simulink model "SVpwm2L_block_level"  (R2023b)
settings: Solver=FixedStepAuto  StartTime=0.0  StopTime=0.1  FixedStep=1e-5  RelTol=1e-4  EnableMultiTasking=on
libraries: spsIGBTDiodeLib x6, spsSeriesRLCBranchLib x3, spsVoltageMeasurementLib x2, spsDCVoltageSourceLib x1, spsGroundLib x1, simulink x1, spsThreePhaseVIMeasurementLib x1, sps_lib x1
settings Model: Creator=Ranit  LastModifiedBy=hhp
settings SolverCC: AlgebraicLoopSolver=TrustRegion
settings DataIOCC: ReturnWorkspaceOutputs=off
settings OptimizationCC: LifeSpan=inf
settings DebuggingCC: UnconnectedInputMsg=warning  UnconnectedOutputMsg=warning  UnconnectedLineMsg=warning  SFUnexpectedBacktrackingDiag=warning  SFNoUnconditionalDefaultTransitionDiag=warning  ArithmeticOperatorsInVariantConditions=warning
settings ModelReferenceCC: EnableRefExpFcnMdlSchedulingChecks=on
settings SFSimCC: SimUseLocalCustomCode=off  CustomCodeUndefinedFunction=UseInterfaceOnly
settings RTWCC: RTWUseLocalCustomCode=off
settings CodeAppCC: StateflowObjectComments=on
settings GRTTargetCC: TargetLangStandard=C89/C90 (ANSI)
settings ConfigComp: CovMetricSettings=dw  CovSaveCumulativeToWorkspaceVar=on  CovSaveSingleToWorkspaceVar=on  CovExternalEMLEnable=off
settings SimscapeCC: SimscapeNormalizeSystem=off

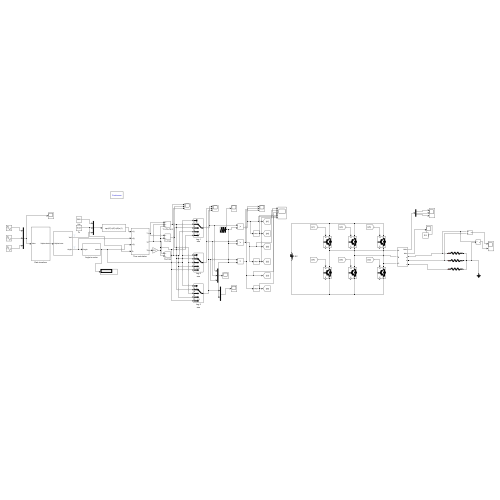
[thumbnail: Simulink's stored preview of the top-level diagram]
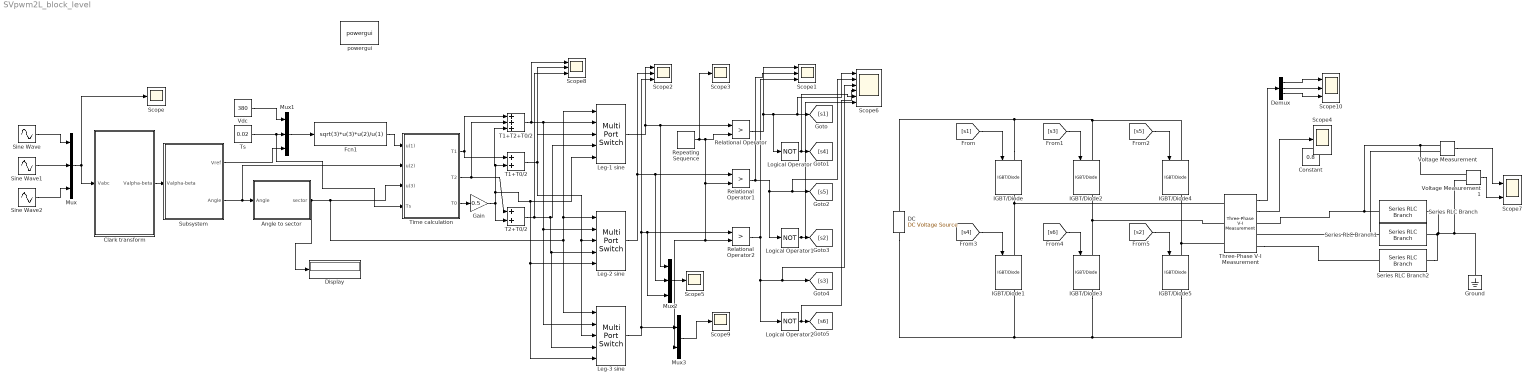
== system SVpwm2L_block_level ==
  Angle to sector : Subsystem
  Clark transform : Subsystem
  Constant : Constant  Value=0.8
  "DC " : spsDCVoltageSourceLib/DC Voltage Source  Amplitude=400  Measurements=None
  Demux : Demux  Outputs=3
  Display : Display
  Fcn1 : Fcn  Expr=sqrt(3)*u(3)*u(2)/u(1)
  Gain : Gain  Gain=0.5
  Ground : spsGroundLib/Ground  LConnTagsString=a
  IGBT/Diode{,1..5} (6 alike) : spsIGBTDiodeLib/IGBT//Diode  Ron=1e-3  Rs=1e5  Cs=inf  Measurements=on
  Leg-1 sine : MultiPortSwitch  DataPortOrder=Specify indices  Inputs=4  DataPortIndices={[1,6],2,5,[3,4]}  SaturateOnIntegerOverflow=off  InputSameDT=off
  Leg-2 sine : MultiPortSwitch  DataPortOrder=Specify indices  Inputs=4  DataPortIndices={[2,3],4,1,[5,6]}  SaturateOnIntegerOverflow=off  InputSameDT=off
  Leg-3 sine : MultiPortSwitch  DataPortOrder=Specify indices  Inputs=4  DataPortIndices={[4,5],6,3,[1,2]}  SaturateOnIntegerOverflow=off  InputSameDT=off
  Logical Operator : Logic  Operator=NOT  AllPortsSameDT=off  OutDataTypeStr=boolean
  Logical Operator1 : Logic  Operator=NOT  AllPortsSameDT=off  OutDataTypeStr=boolean
  Logical Operator2 : Logic  Operator=NOT  AllPortsSameDT=off  OutDataTypeStr=boolean
  Mux : Mux  Inputs=3
  Mux1 : Mux  Inputs=3
  Mux2 : Mux  Inputs=3
  Mux3 : Mux  Inputs=2
  Relational Operator : RelationalOperator  Operator=>  OutDataTypeStr=boolean  InputSameDT=off
  Relational Operator1 : RelationalOperator  Operator=>  OutDataTypeStr=boolean  InputSameDT=off
  Relational Operator2 : RelationalOperator  Operator=>  OutDataTypeStr=boolean  InputSameDT=off
  Repeating Sequence : simulink/Sources/Repeating Sequence  rep_seq_t=[0 1]*[1/3000]  rep_seq_y=[0 0.03]
  Scope{,3..5,9} (5 alike) : Scope
  Scope{1..2,8,10} (4 alike) : Scope  NumInputPorts=3
  Scope6 : Scope  NumInputPorts=6
  Scope7 : Scope  NumInputPorts=2
  Series RLC Branch : spsSeriesRLCBranchLib/Series RLC Branch  LConnTagsString=__new0  RConnTagsString=__new0  BranchType=R  Resistance=5  Inductance=1e-3  SetiL0=off  InitialCurrent=0  Capacitance=1e-6  Setx0=off  InitialVoltage=0  Measurements=None
  Series RLC Branch1 : spsSeriesRLCBranchLib/Series RLC Branch  LConnTagsString=__new0  RConnTagsString=__new0  BranchType=R  Resistance=5  Inductance=1e-3  SetiL0=off  InitialCurrent=0  Capacitance=1e-6  Setx0=off  InitialVoltage=0  Measurements=None
  Series RLC Branch2 : spsSeriesRLCBranchLib/Series RLC Branch  LConnTagsString=__new0  RConnTagsString=__new0  BranchType=R  Resistance=5  Inductance=1e-3  SetiL0=off  InitialCurrent=0  Capacitance=1e-6  Setx0=off  InitialVoltage=0  Measurements=None
  Sine Wave : Sin  Amplitude=230  Frequency=2*pi*50  SampleTime=0
  Sine Wave1 : Sin  Amplitude=230  Frequency=2*pi*50  Phase=2*pi/3  SampleTime=0
  Sine Wave2 : Sin  Amplitude=230  Frequency=2*pi*50  Phase=4*pi/3  SampleTime=0
  Subsystem : Subsystem
  T1+T0/2 : Sum
  T1+T2+T0/2 : Sum  Inputs=+++
  T2+T0/2 : Sum
  Three-Phase V-I Measurement : spsThreePhaseVIMeasurementLib/Three-Phase V-I Measurement  VoltageMeasurement=phase-to-phase  SetLabelV=off  LabelV=Vabc  Vpu=off  VpuLL=off  CurrentMeasurement=yes  SetLabelI=off  LabelI=Iabc  Ipu=off  Pbase=100e6  Vbase=500e3  OutputType=Complex  PhasorSimulation=off  PSBequivalent=0
  Time calculation : Subsystem
  Ts : Constant  Value=0.02
  Vdc : Constant  Value=380
  Voltage Measurement : spsVoltageMeasurementLib/Voltage Measurement  PhasorSimulation=off  OutputType=Complex  PSBequivalent=0
  Voltage Measurement1 : spsVoltageMeasurementLib/Voltage Measurement  PhasorSimulation=off  OutputType=Complex  PSBequivalent=0
  powergui : sps_lib/powergui  Priority=1  SimulationMode=Continuous  SampleTime=10e-6  frequency=60  Iterations=50  frequencyindice=0  Pbase=100e6  ErrMax=1e-4  UnitsV=kV  UnitsW=MW  buscounter=0  FunctionMessages=off  echomessages=off  EnableUseOfTLC=off  CurrentSourceSwitches=on  DisableSnubberDevices=off  DisableRonSwitches=off  DisableVfSwitches=off  DisplayEquations=off  AutomaticDiscreteSolvers=off  SolverType=Tustin/Backward Euler (TBE)  Interpol=off  ExternalGateDelay=off  methode=off  Ts=10  x0status=blocks  SPID=off  SwTol=0  HookPort=off  NonlinearTolerance=1e-4  nMaxIteration=100  ContinueOnMaxIteration=off  RestoreLinks=warning  ResistiveCurrentMeasurement=off  Frange=[0:2:500]  Ylog=off  Xlog=on  ShowGrid=off  save=off  variable=ZData  structure=ScopeData1  ZoomFFT=off  StartTime=0.0  cycles=1  DisplayStyle=1  fundamental=50  FreqAxis=off  MaxFrequency=1000  frequencyindicesteady=1  RmsSteady=1  display=off
  wires:
  Sine Wave1/1 -> Mux/2
  Mux/1 -> Clark transform/1(Vabc), Scope/1
  Clark transform/1(Valpha-beta) -> Subsystem/1(Valpha-beta)
  Sine Wave/1 -> Mux/1
  Sine Wave2/1 -> Mux/3
  Subsystem/2(Angle) -> Angle to sector/1(Angle), Time calculation/2(u(2))
  Subsystem/1(Vref) -> Mux1/3
  Ts/1 -> Time calculation/4(Ts), Mux1/2
  Vdc/1 -> Mux1/1
  Mux1/1 -> Fcn1/1
  Fcn1/1 -> Time calculation/1(u(1))
  Time calculation/1(T1) -> T1+T2+T0/2/1, T1+T0/2/1
  Time calculation/2(T2) -> T1+T2+T0/2/2, T2+T0/2/1
  Time calculation/3(T0) -> Gain/1
  Gain/1 -> Leg-3 sine/5, Leg-2 sine/5, Leg-1 sine/5, T1+T0/2/2, T1+T2+T0/2/3, T2+T0/2/2
  Leg-1 sine/1 -> Scope2/1, Mux2/1, Relational Operator/1
  Leg-2 sine/1 -> Scope2/2, Mux2/2, Relational Operator1/1
  Leg-3 sine/1 -> Mux2/3, Relational Operator2/1, Scope2/3, Mux3/1
  Angle to sector/1(sector) -> Leg-1 sine/1, Leg-2 sine/1, Leg-3 sine/1, Time calculation/3(u(3)), Display/1
  T1+T2+T0/2/1 -> Scope8/1, Leg-3 sine/2, Leg-2 sine/2, Leg-1 sine/2
  T1+T0/2/1 -> Scope8/2, Leg-3 sine/3, Leg-2 sine/3, Leg-1 sine/3
  T2+T0/2/1 -> Scope8/3, Leg-3 sine/4, Leg-2 sine/4, Leg-1 sine/4
  Repeating Sequence/1 -> Scope3/1, Relational Operator2/2, Mux3/2, Relational Operator1/2, Relational Operator/2
  Relational Operator1/1 -> Scope6/2, [s5], Logical Operator1/1, Scope1/2
  Relational Operator2/1 -> Scope1/3, Logical Operator2/1, Scope6/3, [s3]
  [s2] -> IGBT/Diode5/1
  [s5] -> IGBT/Diode4/1
  [s3] -> IGBT/Diode2/1
  [s1] -> IGBT/Diode/1
  [s4] -> IGBT/Diode1/1
  [s6] -> IGBT/Diode3/1
  Relational Operator/1 -> Scope6/1, [s1], Logical Operator/1, Scope1/1
  Logical Operator/1 -> Scope6/5, [s4]
  Logical Operator1/1 -> Scope6/6, [s2]
  Logical Operator2/1 -> Scope6/4, [s6]
  Mux2/1 -> Scope5/1
  Mux3/1 -> Scope9/1
  Demux/1 -> Scope10/1
  Demux/2 -> Scope10/2
  Demux/3 -> Scope10/3
  Three-Phase V-I Measurement/1 -> Demux/1
  Three-Phase V-I Measurement/2 -> Scope4/1
  Voltage Measurement/1 -> Scope7/1
  Voltage Measurement1/1 -> Scope7/2
  connections:
  IGBT/Diode/LConn1 -- "DC "/RConn1 -- IGBT/Diode4/LConn1 -- IGBT/Diode2/LConn1
  IGBT/Diode1/RConn1 -- "DC "/LConn1 -- IGBT/Diode5/RConn1 -- IGBT/Diode3/RConn1
  IGBT/Diode4/RConn1 -- Three-Phase V-I Measurement/LConn3 -- IGBT/Diode5/LConn1
  Series RLC Branch/LConn1 -- Voltage Measurement1/LConn1 -- Voltage Measurement/LConn1 -- Three-Phase V-I Measurement/RConn1
  Series RLC Branch1/LConn1 -- Voltage Measurement/LConn2 -- Three-Phase V-I Measurement/RConn2
  Three-Phase V-I Measurement/RConn3 -- Series RLC Branch2/LConn1
  IGBT/Diode/RConn1 -- Three-Phase V-I Measurement/LConn1 -- IGBT/Diode1/LConn1
  Three-Phase V-I Measurement/LConn2 -- IGBT/Diode2/RConn1 -- IGBT/Diode3/LConn1
  Series RLC Branch/RConn1 -- Voltage Measurement1/LConn2 -- Ground/LConn1 -- Series RLC Branch2/RConn1 -- Series RLC Branch1/RConn1

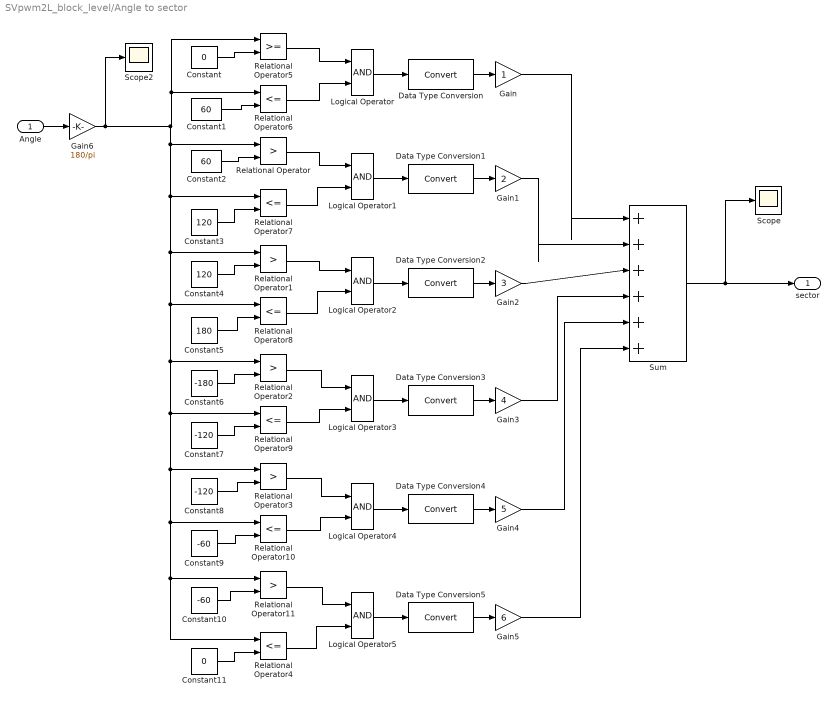
== system SVpwm2L_block_level/Angle to sector ==
  Angle : Inport
  Constant : Constant  Value=0
  Constant1 : Constant  Value=60
  Constant10 : Constant  Value=-60
  Constant11 : Constant  Value=0
  Constant2 : Constant  Value=60
  Constant3 : Constant  Value=120
  Constant4 : Constant  Value=120
  Constant5 : Constant  Value=180
  Constant6 : Constant  Value=-180
  Constant7 : Constant  Value=-120
  Constant8 : Constant  Value=-120
  Constant9 : Constant  Value=-60
  Data Type Conversion{,1..5} (6 alike) : DataTypeConversion  SaturateOnIntegerOverflow=off  RndMeth=Floor
  Gain : Gain
  Gain1 : Gain  Gain=2
  Gain2 : Gain  Gain=3
  Gain3 : Gain  Gain=4
  Gain4 : Gain  Gain=5
  Gain5 : Gain  Gain=6
  Gain6 : Gain  Gain=180/pi
  Logical Operator{,1..5} (6 alike) : Logic  AllPortsSameDT=off  OutDataTypeStr=boolean
  Relational Operator{,1..3,11} (5 alike) : RelationalOperator  Operator=>  OutDataTypeStr=boolean  InputSameDT=off
  Relational Operator{4,6..10} (6 alike) : RelationalOperator  Operator=<=  OutDataTypeStr=boolean  InputSameDT=off
  Relational Operator5 : RelationalOperator  OutDataTypeStr=boolean  InputSameDT=off
  Scope : Scope
  Scope2 : Scope
  Sum : Sum  Inputs=|++++++
  sector : Outport
  wires:
  Constant/1 -> Relational Operator5/2
  Constant1/1 -> Relational Operator6/2
  Constant2/1 -> Relational Operator/2
  Constant3/1 -> Relational Operator7/2
  Constant5/1 -> Relational Operator8/2
  Constant6/1 -> Relational Operator2/2
  Constant7/1 -> Relational Operator9/2
  Constant8/1 -> Relational Operator3/2
  Constant9/1 -> Relational Operator10/2
  Constant10/1 -> Relational Operator11/2
  Constant11/1 -> Relational Operator4/2
  Constant4/1 -> Relational Operator1/2
  Relational Operator11/1 -> Logical Operator5/1
  Relational Operator4/1 -> Logical Operator5/2
  Relational Operator3/1 -> Logical Operator4/1
  Relational Operator10/1 -> Logical Operator4/2
  Relational Operator2/1 -> Logical Operator3/1
  Relational Operator9/1 -> Logical Operator3/2
  Relational Operator5/1 -> Logical Operator/1
  Relational Operator6/1 -> Logical Operator/2
  Relational Operator/1 -> Logical Operator1/1
  Relational Operator7/1 -> Logical Operator1/2
  Relational Operator1/1 -> Logical Operator2/1
  Relational Operator8/1 -> Logical Operator2/2
  Gain4/1 -> Sum/5
  Gain3/1 -> Sum/4
  Gain5/1 -> Sum/6
  Gain2/1 -> Sum/3
  Gain1/1 -> Sum/2
  Gain/1 -> Sum/1
  Sum/1 -> Scope/1, sector/1
  Logical Operator/1 -> Data Type Conversion/1
  Data Type Conversion/1 -> Gain/1
  Data Type Conversion1/1 -> Gain1/1
  Logical Operator1/1 -> Data Type Conversion1/1
  Data Type Conversion2/1 -> Gain2/1
  Logical Operator2/1 -> Data Type Conversion2/1
  Data Type Conversion3/1 -> Gain3/1
  Logical Operator3/1 -> Data Type Conversion3/1
  Data Type Conversion4/1 -> Gain4/1
  Logical Operator4/1 -> Data Type Conversion4/1
  Data Type Conversion5/1 -> Gain5/1
  Logical Operator5/1 -> Data Type Conversion5/1
  Angle/1 -> Gain6/1
  Gain6/1 -> Scope2/1, Relational Operator/1, Relational Operator7/1, Relational Operator1/1, Relational Operator8/1, Relational Operator2/1, Relational Operator10/1, Relational Operator11/1, Relational Operator4/1, Relational Operator3/1, Relational Operator9/1, Relational Operator6/1, Relational Operator5/1

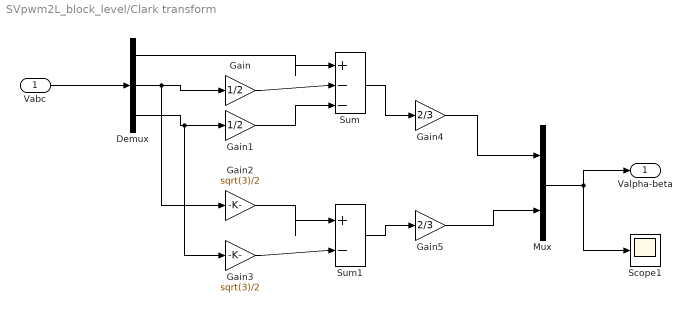
== system SVpwm2L_block_level/Clark transform ==
  Vabc : Inport
  Demux : Demux  Outputs=3
  Gain : Gain  Gain=1/2
  Gain1 : Gain  Gain=1/2
  Gain2 : Gain  Gain=sqrt(3)/2
  Gain3 : Gain  Gain=sqrt(3)/2
  Gain4 : Gain  Gain=2/3
  Gain5 : Gain  Gain=2/3
  Mux : Mux  Inputs=2
  Scope1 : Scope
  Sum : Sum  Inputs=|+--
  Sum1 : Sum  Inputs=|+-
  Valpha-beta : Outport
  wires:
  Vabc/1 -> Demux/1
  Demux/1 -> Sum/1
  Gain/1 -> Sum/2
  Demux/2 -> Gain2/1, Gain/1
  Demux/3 -> Gain3/1, Gain1/1
  Gain1/1 -> Sum/3
  Gain2/1 -> Sum1/1
  Gain3/1 -> Sum1/2
  Mux/1 -> Valpha-beta/1, Scope1/1
  Sum1/1 -> Gain5/1
  Gain5/1 -> Mux/2
  Sum/1 -> Gain4/1
  Gain4/1 -> Mux/1

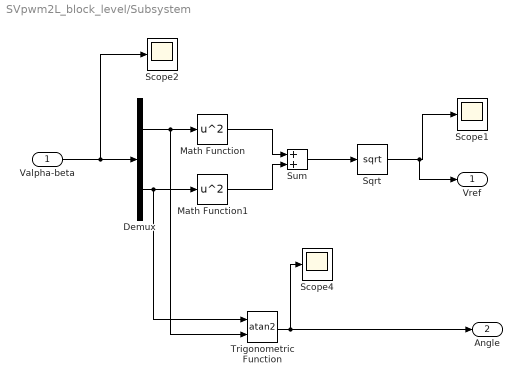
== system SVpwm2L_block_level/Subsystem ==
  Valpha-beta : Inport
  Demux : Demux  Outputs=2
  Math Function : Math  Operator=square  SignedPower=on
  Math Function1 : Math  Operator=square  SignedPower=on
  Scope1 : Scope
  Scope2 : Scope
  Scope4 : Scope
  Sqrt : Sqrt
  Sum : Sum  Inputs=|++
  Trigonometric Function : Trigonometry  Operator=atan2
  Vref : Outport
  Angle : Outport  Port=2
  wires:
  Valpha-beta/1 -> Scope2/1, Demux/1
  Demux/1 -> Trigonometric Function/2, Math Function/1
  Demux/2 -> Trigonometric Function/1, Math Function1/1
  Math Function/1 -> Sum/1
  Math Function1/1 -> Sum/2
  Sum/1 -> Sqrt/1
  Sqrt/1 -> Vref/1, Scope1/1
  Trigonometric Function/1 -> Scope4/1, Angle/1

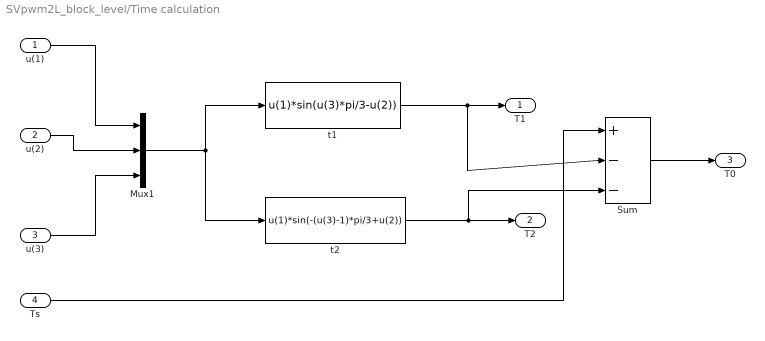
== system SVpwm2L_block_level/Time calculation ==
  u(1) : Inport
  u(2) : Inport  Port=2
  u(3) : Inport  Port=3
  Ts : Inport  Port=4
  Mux1 : Mux  Inputs=3
  Sum : Sum  Inputs=|+--
  t1 : Fcn  Expr=u(1)*sin(u(3)*pi/3-u(2))
  t2 : Fcn  Expr=u(1)*sin(-(u(3)-1)*pi/3+u(2))
  T1 : Outport
  T2 : Outport  Port=2
  T0 : Outport  Port=3
  wires:
  u(1)/1 -> Mux1/1
  u(2)/1 -> Mux1/2
  u(3)/1 -> Mux1/3
  Mux1/1 -> t2/1, t1/1
  t1/1 -> Sum/2, T1/1
  t2/1 -> Sum/3, T2/1
  Ts/1 -> Sum/1
  Sum/1 -> T0/1
